simulink model "PMSM_SMO_dq"  (Simulink 9.3)
settings: Solver=ode3  StartTime=0.0  StopTime=1  FixedStep=Ts  RelTol=1e-3  EnableMultiTasking=on
InitFcn:
  | Ts = 10e-6;
  | 
  | Ra = 0.011;
  | Ld = 0.0016;
  | Lq = 0.001;
  | flux =0.077;
  | 
  | m0 = 2;
  | ksild = 700;
  | A = exp(-Ra/Ld*Ts);
  | B = (1-A)/Ra;
  | Aq = exp(-Ra/Lq*Ts);
  | Bq = (1-Aq)/Ra;
undefined symbols (not defined in the file or in its folder): DiscIntNeverNeededParam
libraries: powerlib_extras x9, powerlib x5, simulink x1
settings Model: Creator=Administrator  LastModifiedBy=Administrator
settings DataIOCC: LimitDataPoints=on
settings OptimizationCC: ExpressionDepthLimit=2147483647  InitFltsAndDblsToZero=on
settings DebuggingCC: SaveWithParameterizedLinksMsg=none  SolverPrmCheckMsg=warning  StateNameClashWarn=warning
settings GRTTargetCC: TargetFcnLib=ansi_tfl_tmw.mat  GeneratePreprocessorConditionals=Disable all
settings ConfigComp: CovSFcnEnable=off
settings SimscapeCC: SimscapeNormalizeSystem=off

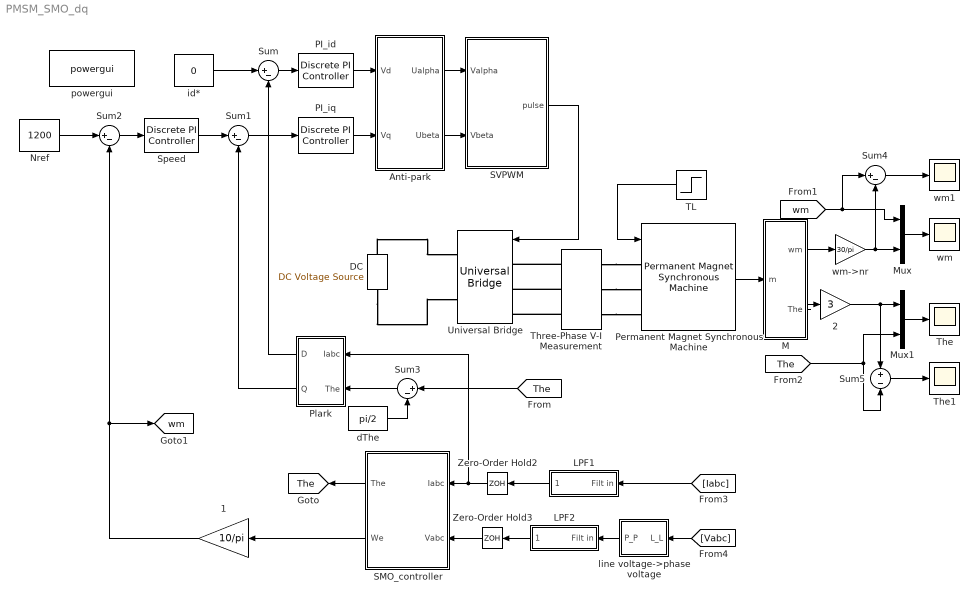
== system PMSM_SMO_dq ==
  1 : Gain  Gain=10/pi
  2 : Gain  Gain=3
  Anti-park : Subsystem
  "DC " : powerlib/Electrical Sources/DC Voltage Source  Amplitude=311  Measurements=None
      settings: SourceProductName=Simscape Electrical
  LPF1 : Subsystem  mask{wcc=3000, Ts=Ts}
      mask prompts: wcc "Control Filter cutoff frequency(Hz):"; Ts "sampling time"
  LPF2 : Subsystem  mask{wcc=3000, Ts=Ts}
      mask prompts: wcc "Control Filter cutoff frequency(Hz):"; Ts "sampling time"
  M : Subsystem
  Mux : Mux  Inputs=2
  Mux1 : Mux  Inputs=2
  Nref : Constant  Value=1200
  "PI_id " : powerlib_extras/Discrete  Control Blocks/Discrete PI Controller  Kp=0.0016*20000  Ki=0.011*20000  Par_Limits=[250 -250]  Init=0  Ts=Ts
      settings: SourceProductName=Simscape Electrical
  PI_iq : powerlib_extras/Discrete  Control Blocks/Discrete PI Controller  Kp=0.001*20000  Ki=0.011*20000  Par_Limits=[250 -250]  Init=0  Ts=Ts
      settings: SourceProductName=Simscape Electrical
  Permanent Magnet Synchronous Machine : powerlib/Machines/Permanent Magnet Synchronous Machine  NbPhases=3  FluxDistribution=Sinusoidal  RotorType=Salient-pole  MechanicalLoad=Torque Tm  PresetModel=No  ShowDetailedParameters=on  MeasurementBus=off  Resistance=0.011  Inductance=8.5e-3  dqInductances=[0.0016,0.001]  La=0.000835  MachineConstant=Flux linkage established by magnets (V.s)  Flux=0.077  VoltageCst=41.8988  TorqueCst=0.3465  Flat=120  Mechanical=[0.0008 0 3]  PolePairs=3  InitialConditions=[0,0, 0,0]  InitialConditions5ph=[0 0 0 0 0 0]  TsPowergui=0  TsBlock=-1  RefAngle=90 degrees behind phase A axis (modified Park)
  Plark : Subsystem
  SMO_controller : Subsystem  mask{Ts=Ts}
  SVPWM : Subsystem
  "Speed " : powerlib_extras/Discrete  Control Blocks/Discrete PI Controller  Kp=0.02  Ki=1  Par_Limits=[300 -300]  Init=0  Ts=Ts
      settings: SourceProductName=Simscape Electrical
  Sum{,1..4} (5 alike) : Sum  Inputs=|+-
  Sum5 : Sum  Inputs=+|-
  TL : Step  Time=0.5  After=1*0  SampleTime=0
  The : Scope
  The1 : Scope
  Three-Phase V-I Measurement : powerlib/Measurements/Three-Phase V-I Measurement  VoltageMeasurement=phase-to-phase  SetLabelV=on  LabelV=Vabc  Vpu=off  VpuLL=off  CurrentMeasurement=yes  SetLabelI=on  LabelI=Iabc  Ipu=off  Pbase=100e6  Vbase=500e3  OutputType=Complex  PhasorSimulation=off  PSBequivalent=0
      settings: SourceProductName=Simscape Electrical
  Universal Bridge : powerlib/Power Electronics/Universal Bridge  Arms=3  SnubberResistance=1e5  SnubberCapacitance=inf  Device=IGBT / Diodes  Ron=1e-3  Lon=0  ForwardVoltages="[  0  0  ]"  ForwardVoltage=0  GTOparameters=[ 10e-6 , 20e-6 ]  IGBTparameters=[ 1e-6 , 2e-6 ]  Measurements=None  Measurements_2=None  converterType=Rectifier
      settings: SourceProductName=Simscape Electrical
  Zero-Order Hold2 : ZeroOrderHold  SampleTime=Ts
  Zero-Order Hold3 : ZeroOrderHold  SampleTime=Ts
  dThe : Constant  Value=pi/2
  id* : Constant  Value=0
  line voltage->phase voltage : Subsystem
  powergui : powerlib/powergui  SimulationMode=Discrete  SampleTime=Ts  frequency=60  Iterations=50  frequencyindice=0  Pbase=100e6  ErrMax=1e-4  UnitsV=kV  UnitsW=MW  buscounter=0  FunctionMessages=off  echomessages=off  EnableUseOfTLC=off  CurrentSourceSwitches=off  DisableSnubberDevices=off  DisableRonSwitches=off  DisableVfSwitches=off  DisplayEquations=off  AutomaticDiscreteSolvers=off  SolverType=Tustin/Backward Euler (TBE)  Interpol=off  ExternalGateDelay=off  methode=off  Ts=0  x0status=blocks  SPID=off  SwTol=0  HookPort=off  NonlinearTolerance=0  nMaxIteration=15  ContinueOnMaxIteration=off  RestoreLinks=warning  ResistiveCurrentMeasurement=off  Frange=[0:2:500]  Ylog=off  Xlog=on  ShowGrid=off  save=off  variable=ZData  structure=0  ZoomFFT=off  StartTime=0.0  cycles=1  DisplayStyle=1  fundamental=60  FreqAxis=off  MaxFrequency=1000  frequencyindicesteady=1  RmsSteady=1  display=off
      settings: SourceProductName=Simscape Electrical
  wm : Scope
  wm->nr : Gain  Gain=30/pi
  wm1 : Scope
  tag scope: The=global, wm=global
  wires:
  SVPWM/1(pulse) -> Universal Bridge/1
  Permanent Magnet Synchronous Machine/1 -> M/1(m)
  "PI_id "/1 -> Anti-park/1(Vd)
  PI_iq/1 -> Anti-park/2(Vq)
  Sum/1 -> "PI_id "/1
  Sum1/1 -> PI_iq/1
  Sum2/1 -> "Speed "/1
  Nref/1 -> Sum2/1
  "Speed "/1 -> Sum1/1
  1/1 -> [wm], Sum2/2
  Anti-park/1(Ualpha) -> SVPWM/1(Valpha)
  Anti-park/2(Ubeta) -> SVPWM/2(Vbeta)
  TL/1 -> Permanent Magnet Synchronous Machine/1
  M/1(wm) -> wm->nr/1
  id*/1 -> Sum/1
  Plark/1(D) -> Sum/2
  Plark/2(Q) -> Sum1/2
  dThe/1 -> Sum3/2
  Sum3/1 -> Plark/2(The)
  M/2(The) -> 2/1
  LPF2/1(Filt out) -> Zero-Order Hold3/1
  Zero-Order Hold3/1 -> SMO_controller/2(Vabc)
  Zero-Order Hold2/1 -> Plark/1(Iabc), SMO_controller/1(Iabc)
  LPF1/1(Filt out) -> Zero-Order Hold2/1
  SMO_controller/1(The) -> [The]
  [The] -> Sum3/1
  wm->nr/1 -> Mux/2, Sum4/2
  [wm] -> Mux/1, Sum4/1
  Mux/1 -> wm/1
  Sum4/1 -> wm1/1
  2/1 -> Sum5/1, Mux1/1
  Mux1/1 -> The/1
  [The] -> Mux1/2, Sum5/2
  Sum5/1 -> The1/1
  [Iabc] -> LPF1/1(Filt in)
  [Vabc] -> line voltage->phase voltage/1(L_L)
  line voltage->phase voltage/1(P_P) -> LPF2/1(Filt in)
  SMO_controller/2(We) -> 1/1
  connections:
  "DC "/RConn1 -- Universal Bridge/RConn1
  "DC "/LConn1 -- Universal Bridge/RConn2
  Three-Phase V-I Measurement/LConn1 -- Universal Bridge/LConn1
  Three-Phase V-I Measurement/RConn1 -- Permanent Magnet Synchronous Machine/LConn1
  Three-Phase V-I Measurement/LConn2 -- Universal Bridge/LConn2
  Three-Phase V-I Measurement/LConn3 -- Universal Bridge/LConn3
  Three-Phase V-I Measurement/RConn2 -- Permanent Magnet Synchronous Machine/LConn2
  Three-Phase V-I Measurement/RConn3 -- Permanent Magnet Synchronous Machine/LConn3

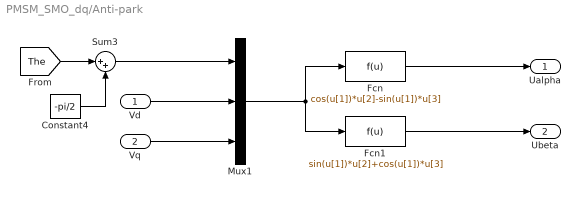
== system PMSM_SMO_dq/Anti-park ==
  Vd : Inport
  Vq : Inport  Port=2
  Constant4 : Constant  Value=-pi/2
  Fcn : Fcn  Expr=cos(u[1])*u[2]-sin(u[1])*u[3]
  Fcn1 : Fcn  Expr=sin(u[1])*u[2]+cos(u[1])*u[3]
  Mux1 : Mux  Inputs=3
  Sum3 : Sum  Inputs=|++
  Ualpha : Outport
  Ubeta : Outport  Port=2
  wires:
  Fcn1/1 -> Ubeta/1
  Fcn/1 -> Ualpha/1
  Mux1/1 -> Fcn/1, Fcn1/1
  Vd/1 -> Mux1/2
  Vq/1 -> Mux1/3
  Sum3/1 -> Mux1/1
  [The] -> Sum3/1
  Constant4/1 -> Sum3/2

== system PMSM_SMO_dq/LPF1 ==
  Filt in : Inport
  Demux1 : Demux  Outputs=3
  LPF1 : powerlib_extras/Discrete  Control Blocks/Discrete 1st-Order Filter  FilterType=Lowpass  Tc=1/(2*pi*wcc)  Ts=Ts  Initialize=off  Vac_Init=[0.8 -25 60]  Vdc_Init=-0.4  PlotResponse=off  param1=[1 500 1]
      settings: SourceProductName=Simscape Electrical  SourceProductBaseCode=PS
  LPF2 : powerlib_extras/Discrete  Control Blocks/Discrete 1st-Order Filter  FilterType=Lowpass  Tc=1/(2*pi*wcc)  Ts=Ts  Initialize=off  Vac_Init=[0.8 -25 60]  Vdc_Init=-0.4  PlotResponse=off  param1=[1 500 1]
      settings: SourceProductName=Simscape Electrical  SourceProductBaseCode=PS
  LPF3 : powerlib_extras/Discrete  Control Blocks/Discrete 1st-Order Filter  FilterType=Lowpass  Tc=1/(2*pi*wcc)  Ts=Ts  Initialize=off  Vac_Init=[0.8 -25 60]  Vdc_Init=-0.4  PlotResponse=off  param1=[1 4000 1]
      settings: SourceProductName=Simscape Electrical  SourceProductBaseCode=PS
  Mux1 : Mux  Inputs=3
  Filt out : Outport
  wires:
  Demux1/1 -> LPF1/1
  LPF1/1 -> Mux1/1
  Demux1/2 -> LPF2/1
  LPF2/1 -> Mux1/2
  Filt in/1 -> Demux1/1
  Mux1/1 -> Filt out/1
  Demux1/3 -> LPF3/1
  LPF3/1 -> Mux1/3

== system PMSM_SMO_dq/LPF2 ==
  Filt in : Inport
  Demux1 : Demux  Outputs=3
  LPF1 : powerlib_extras/Discrete  Control Blocks/Discrete 1st-Order Filter  FilterType=Lowpass  Tc=1/(2*pi*wcc)  Ts=Ts  Initialize=off  Vac_Init=[0.8 -25 60]  Vdc_Init=-0.4  PlotResponse=off  param1=[1 500 1]
      settings: SourceProductName=Simscape Electrical  SourceProductBaseCode=PS
  LPF2 : powerlib_extras/Discrete  Control Blocks/Discrete 1st-Order Filter  FilterType=Lowpass  Tc=1/(2*pi*wcc)  Ts=Ts  Initialize=off  Vac_Init=[0.8 -25 60]  Vdc_Init=-0.4  PlotResponse=off  param1=[1 500 1]
      settings: SourceProductName=Simscape Electrical  SourceProductBaseCode=PS
  LPF3 : powerlib_extras/Discrete  Control Blocks/Discrete 1st-Order Filter  FilterType=Lowpass  Tc=1/(2*pi*wcc)  Ts=Ts  Initialize=off  Vac_Init=[0.8 -25 60]  Vdc_Init=-0.4  PlotResponse=off  param1=[1 4000 1]
      settings: SourceProductName=Simscape Electrical  SourceProductBaseCode=PS
  Mux1 : Mux  Inputs=3
  Filt out : Outport
  wires:
  LPF3/1 -> Mux1/3
  Demux1/3 -> LPF3/1
  Mux1/1 -> Filt out/1
  Filt in/1 -> Demux1/1
  LPF2/1 -> Mux1/2
  Demux1/2 -> LPF2/1
  LPF1/1 -> Mux1/1
  Demux1/1 -> LPF1/1

== system PMSM_SMO_dq/M ==
  m : Inport
  Bus Selector1 : BusSelector  OutputSignals=Rotor speed wm (rad/s),Rotor angle thetam (rad),Electromagnetic torque Te (N*m)
  Terminator : Terminator
  wm : Outport
  The : Outport  Port=2
  wires:
  Bus Selector1/1 -> wm/1  "<Rotor speed wm (rad/s)>"
  Bus Selector1/2 -> The/1  "<Rotor angle thetam (rad)>"
  Bus Selector1/3 -> Terminator/1  "<Electromagnetic torque Te (N*m)>"
  m/1 -> Bus Selector1/1

== system PMSM_SMO_dq/Plark ==
  Iabc : Inport
  The : Inport  Port=2
  Mux : Mux  Inputs=2
  d : Fcn  Expr=(u(1)*cos(u(4))+u(2)*cos(u(4)-2/3*pi)+u(3)*cos(u(4)+2/3*pi))*2/3
  q : Fcn  Expr=-(u(1)*sin(u(4))+u(2)*sin(u(4)-2/3*pi)+u(3)*sin(u(4)+2/3*pi))*2/3
  D : Outport
  Q : Outport  Port=2
  wires:
  Mux/1 -> d/1, q/1
  Iabc/1 -> Mux/1
  d/1 -> D/1
  The/1 -> Mux/2
  q/1 -> Q/1

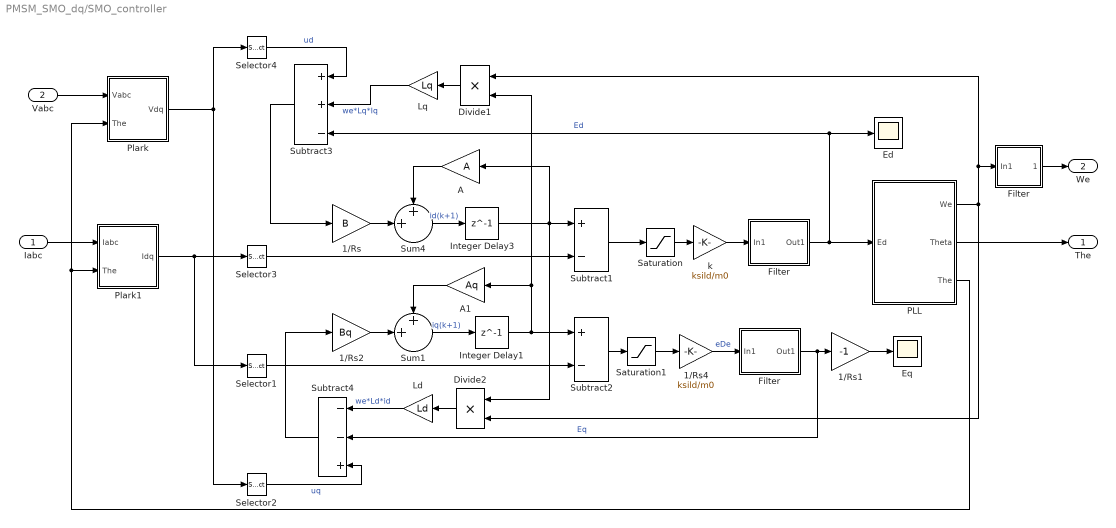
== system PMSM_SMO_dq/SMO_controller ==
  Iabc : Inport
  Vabc : Inport  Port=2
  " Filter" : Subsystem  mask{a=0.97}
  1/Rs : Gain  Gain=B
  1/Rs1 : Gain  Gain=-1
  1/Rs2 : Gain  Gain=Bq
  1/Rs4 : Gain  Gain=ksild/m0
  A : Gain  Gain=A
  A1 : Gain  Gain=Aq
  Divide1 : Product  Inputs=**
  Divide2 : Product  Inputs=**
  Ed : Scope
  Eq : Scope
  "Filter " : Subsystem  mask{a=0.97}
  "Filter  " : Subsystem  mask{a=0.99}
  Integer Delay1 : Delay  DelayLength=1  SampleTime=Ts
  Integer Delay3 : Delay  DelayLength=1  SampleTime=Ts
  Ld : Gain  Gain=Ld
  Lq : Gain  Gain=Lq
  PLL : Subsystem
  Plark : Subsystem
  Plark1 : Subsystem
  Saturation : Saturate  UpperLimit=m0  LowerLimit=-m0
  Saturation1 : Saturate  UpperLimit=m0  LowerLimit=-m0
  Selector1 : Selector  InputPortWidth=2  IndexOptions=Index vector (dialog)  Indices=[2 ]  OutputSizes=1
  Selector2 : Selector  InputPortWidth=2  IndexOptions=Index vector (dialog)  Indices=[2 ]  OutputSizes=1
  Selector3 : Selector  InputPortWidth=2  IndexOptions=Index vector (dialog)  Indices=[1 ]  OutputSizes=1
  Selector4 : Selector  InputPortWidth=2  IndexOptions=Index vector (dialog)  Indices=[1 ]  OutputSizes=1
  Subtract1 : Sum  Inputs=+-
  Subtract2 : Sum  Inputs=+-
  Subtract3 : Sum  Inputs=++-
  Subtract4 : Sum  Inputs=--+
  Sum1 : Sum  Inputs=++|
  Sum4 : Sum  Inputs=++|
  k : Gain  Gain=ksild/m0
  The : Outport
  We : Outport  Port=2
  wires:
  Iabc/1 -> Plark1/1(Iabc)
  Vabc/1 -> Plark/1(Vabc)
  Plark1/1(Idq) -> Selector1/1, Selector3/1
  Plark/1(Vdq) -> Selector4/1, Selector2/1
  Lq/1 -> Subtract3/2  "we*Lq*Iq"
  Saturation/1 -> k/1
  Divide1/1 -> Lq/1
  Sum4/1 -> Integer Delay3/1  "id(k+1)"
  Subtract1/1 -> Saturation/1
  k/1 -> "Filter "/1(In1)
  Subtract3/1 -> 1/Rs/1
  Selector4/1 -> Subtract3/1  "ud"
  1/Rs/1 -> Sum4/2
  A/1 -> Sum4/1
  Selector3/1 -> Subtract1/2
  "Filter "/1(Out1) -> Ed/1, Subtract3/3, PLL/1(Ed)  "Ed"
  Saturation1/1 -> 1/Rs4/1
  Divide2/1 -> Ld/1
  Sum1/1 -> Integer Delay1/1  "iq(k+1)"
  Subtract2/1 -> Saturation1/1
  1/Rs4/1 -> " Filter"/1(In1)  "eDe"
  Subtract4/1 -> 1/Rs2/1
  1/Rs2/1 -> Sum1/2
  " Filter"/1(Out1) -> 1/Rs1/1, Subtract4/2  "Eq"
  A1/1 -> Sum1/1
  Selector1/1 -> Subtract2/2
  Integer Delay1/1 -> Subtract2/1, Divide1/2, A1/1
  Ld/1 -> Subtract4/1  "we*Ld*id"
  Selector2/1 -> Subtract4/3  "uq"
  Integer Delay3/1 -> Subtract1/1, A/1, Divide2/1
  PLL/3(The) -> Plark/2(The), Plark1/2(The)
  PLL/1(We) -> Divide1/1, "Filter  "/1(In1), Divide2/2
  PLL/2(Theta) -> The/1
  "Filter  "/1(Out1) -> We/1
  1/Rs1/1 -> Eq/1

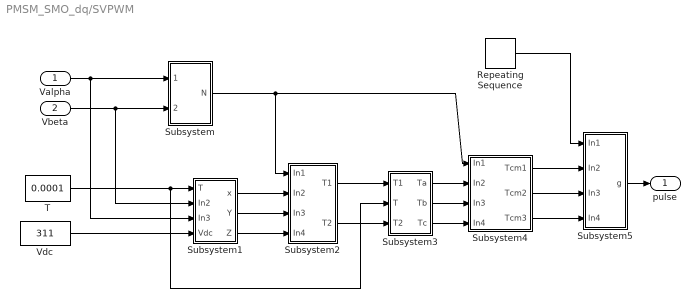
== system PMSM_SMO_dq/SVPWM ==
  Valpha : Inport
  Vbeta : Inport  Port=2
  Repeating Sequence : simulink/Sources/Repeating Sequence  rep_seq_t=[0 0.00005 0.0001]  rep_seq_y=[0 0.00005 0]
  Subsystem : Subsystem
  Subsystem1 : Subsystem
  Subsystem2 : Subsystem
  Subsystem3 : Subsystem
  Subsystem4 : Subsystem
  Subsystem5 : Subsystem
  T : Constant  Value=0.0001
  Vdc : Constant  Value=311
  pulse : Outport
  wires:
  Subsystem5/1(g) -> pulse/1
  Repeating Sequence/1 -> Subsystem5/1(In1)
  Subsystem4/3(Tcm3) -> Subsystem5/4(In4)
  Subsystem4/2(Tcm2) -> Subsystem5/3(In3)
  Subsystem4/1(Tcm1) -> Subsystem5/2(In2)
  Subsystem3/3(Tc) -> Subsystem4/4(In4)
  Subsystem3/2(Tb) -> Subsystem4/3(In3)
  Subsystem3/1(Ta) -> Subsystem4/2(In2)
  Subsystem2/2(T2) -> Subsystem3/3(T2)
  Subsystem2/1(T1) -> Subsystem3/1(T1)
  Subsystem1/3(Z) -> Subsystem2/4(In4)
  Subsystem1/2(Y) -> Subsystem2/3(In3)
  Subsystem1/1(x) -> Subsystem2/2(In2)
  Subsystem/1(N) -> Subsystem4/1(In1), Subsystem2/1(In1)
  Vdc/1 -> Subsystem1/4(Vdc)
  T/1 -> Subsystem3/2(T), Subsystem1/1(T)
  Vbeta/1 -> Subsystem1/2(In2), Subsystem/2(Vbeta)
  Valpha/1 -> Subsystem1/3(In3), Subsystem/1(Valpha)

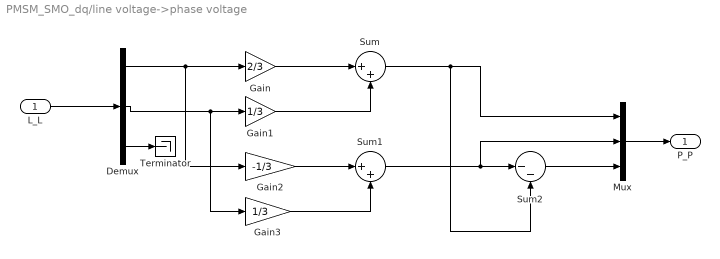
== system PMSM_SMO_dq/line voltage->phase voltage ==
  L_L : Inport
  Demux : Demux  Outputs=3
  Gain : Gain  Gain=2/3
  Gain1 : Gain  Gain=1/3
  Gain2 : Gain  Gain=-1/3
  Gain3 : Gain  Gain=1/3
  Mux : Mux  Inputs=3
  Sum : Sum  Inputs=|++
  Sum1 : Sum  Inputs=|++
  Sum2 : Sum  Inputs=|--
  Terminator : Terminator
  P_P : Outport
  wires:
  Demux/2 -> Gain3/1, Gain1/1
  Demux/1 -> Gain2/1, Gain/1
  Gain/1 -> Sum/1
  Gain1/1 -> Sum/2
  Gain2/1 -> Sum1/1
  Gain3/1 -> Sum1/2
  Sum/1 -> Sum2/2, Mux/1
  Sum2/1 -> Mux/3
  Sum1/1 -> Mux/2, Sum2/1
  Mux/1 -> P_P/1
  L_L/1 -> Demux/1
  Demux/3 -> Terminator/1

== system PMSM_SMO_dq/SMO_controller/ Filter ==
  In1 : Inport
  1/Ld1 : Gain  Gain=a
  1/Ld4 : Gain  Gain=1-a  SampleTime=Ts
  Integer Delay5 : Delay  DelayLength=1  SampleTime=Ts
  Subtract3 : Sum
  Out1 : Outport
  wires:
  In1/1 -> 1/Ld4/1
  1/Ld1/1 -> Subtract3/2
  1/Ld4/1 -> Subtract3/1
  Integer Delay5/1 -> 1/Ld1/1
  Subtract3/1 -> Out1/1, Integer Delay5/1

== system PMSM_SMO_dq/SMO_controller/Filter  ==
  In1 : Inport
  1/Ld1 : Gain  Gain=a
  1/Ld4 : Gain  Gain=1-a  SampleTime=Ts
  Integer Delay5 : Delay  DelayLength=1  SampleTime=Ts
  Subtract3 : Sum
  Out1 : Outport
  wires:
  In1/1 -> 1/Ld4/1
  1/Ld1/1 -> Subtract3/2
  1/Ld4/1 -> Subtract3/1
  Integer Delay5/1 -> 1/Ld1/1
  Subtract3/1 -> Out1/1, Integer Delay5/1

== system PMSM_SMO_dq/SMO_controller/Filter   ==
  In1 : Inport
  1/Ld1 : Gain  Gain=a
  1/Ld4 : Gain  Gain=1-a  SampleTime=Ts
  Integer Delay5 : Delay  DelayLength=1  SampleTime=Ts
  Subtract3 : Sum
  Out1 : Outport
  wires:
  Subtract3/1 -> Integer Delay5/1, Out1/1
  Integer Delay5/1 -> 1/Ld1/1
  1/Ld4/1 -> Subtract3/1
  1/Ld1/1 -> Subtract3/2
  In1/1 -> 1/Ld4/1

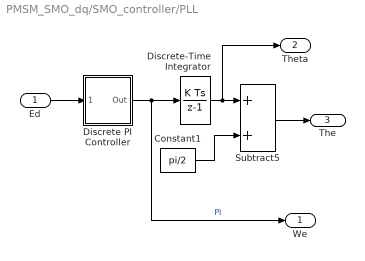
== system PMSM_SMO_dq/SMO_controller/PLL ==
  Ed : Inport
  Constant1 : Constant  Value=pi/2
  Discrete PI Controller : Subsystem  AncestorBlock=|  mask(Discrete PI Controller){Kp=30, Ki=225*2, Par_Limits=[1000 -1000], Init=0, Ts=Ts}
      | powerlib_extras/Discrete 
      | Control Blocks/Discrete
      | PI Controller
      mask prompts: Kp "Proportional gain (Kp):"; Ki "Integral gain (Ki):"; Par_Limits "Output limits: [ Upper   Lower ]"; Init "Output initial value:"; Ts "Sample time:"
      mask help: This block implements a discrete PI controller.
      mask init:
      | UpperLimit=Par_Limits(1);
      | LowerLimit=Par_Limits(2);
      | power_initmask();
      settings: OpenFcn=power_openblockproxy();
      mask Display: disp('PI');
  Discrete-Time Integrator : DiscreteIntegrator  SampleTime=Ts  ICPrevOutput=DiscIntNeverNeededParam  ICPrevScaledInput=DiscIntNeverNeededParam
  Subtract5 : Sum
  We : Outport
  Theta : Outport  Port=2
  The : Outport  Port=3
  wires:
  Discrete-Time Integrator/1 -> Theta/1, Subtract5/1
  Subtract5/1 -> The/1
  Constant1/1 -> Subtract5/2
  Discrete PI Controller/1(Out) -> We/1, Discrete-Time Integrator/1  "PI"
  Ed/1 -> Discrete PI Controller/1(Error)

== system PMSM_SMO_dq/SMO_controller/Plark ==
  Vabc : Inport
  The : Inport  Port=2
  Mux : Mux  Inputs=2
  Mux1 : Mux  Inputs=2
  d : Fcn  Expr=(u(1)*cos(u(4))+u(2)*cos(u(4)-2/3*pi)+u(3)*cos(u(4)+2/3*pi))*2/3
  q : Fcn  Expr=-(u(1)*sin(u(4))+u(2)*sin(u(4)-2/3*pi)+u(3)*sin(u(4)+2/3*pi))*2/3
  Vdq : Outport
  wires:
  Mux/1 -> q/1, d/1
  Vabc/1 -> Mux/1
  The/1 -> Mux/2
  d/1 -> Mux1/1
  q/1 -> Mux1/2
  Mux1/1 -> Vdq/1

== system PMSM_SMO_dq/SMO_controller/Plark1 ==
  Iabc : Inport
  The : Inport  Port=2
  Mux : Mux  Inputs=2
  Mux1 : Mux  Inputs=2
  d : Fcn  Expr=(u(1)*cos(u(4))+u(2)*cos(u(4)-2/3*pi)+u(3)*cos(u(4)+2/3*pi))*2/3
  q : Fcn  Expr=-(u(1)*sin(u(4))+u(2)*sin(u(4)-2/3*pi)+u(3)*sin(u(4)+2/3*pi))*2/3
  Idq : Outport
  wires:
  Mux1/1 -> Idq/1
  q/1 -> Mux1/2
  d/1 -> Mux1/1
  The/1 -> Mux/2
  Iabc/1 -> Mux/1
  Mux/1 -> d/1, q/1

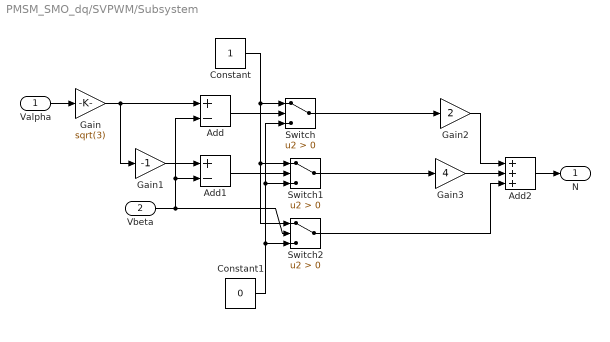
== system PMSM_SMO_dq/SVPWM/Subsystem ==
  Valpha : Inport
  Vbeta : Inport  Port=2
  Add : Sum  Inputs=+-
  Add1 : Sum  Inputs=+-
  Add2 : Sum  Inputs=+++
  Constant : Constant
  Constant1 : Constant  Value=0
  Gain : Gain  Gain=sqrt(3)
  Gain1 : Gain  Gain=-1
  Gain2 : Gain  Gain=2
  Gain3 : Gain  Gain=4
  Switch : Switch  Criteria=u2 > Threshold
  Switch1 : Switch  Criteria=u2 > Threshold
  Switch2 : Switch  Criteria=u2 > Threshold
  N : Outport
  wires:
  Add2/1 -> N/1
  Valpha/1 -> Gain/1
  Gain3/1 -> Add2/2
  Gain2/1 -> Add2/1
  Add1/1 -> Switch1/2
  Gain1/1 -> Add1/1
  Switch1/1 -> Gain3/1
  Switch2/1 -> Add2/3
  Switch/1 -> Gain2/1
  Add/1 -> Switch/2
  Gain/1 -> Gain1/1, Add/1
  Constant1/1 -> Switch/3, Switch1/3, Switch2/3
  Constant/1 -> Switch1/1, Switch2/1, Switch/1
  Vbeta/1 -> Add1/2, Add/2, Switch2/2

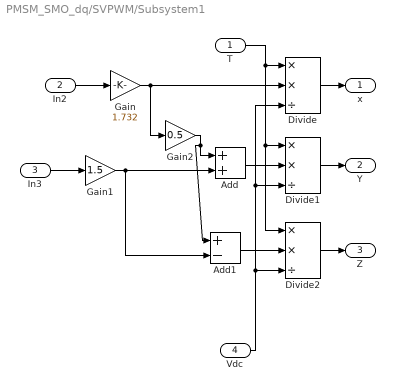
== system PMSM_SMO_dq/SVPWM/Subsystem1 ==
  T : Inport
  In2 : Inport  Port=2
  In3 : Inport  Port=3
  Vdc : Inport  Port=4
  Add : Sum
  Add1 : Sum  Inputs=+-
  Divide : Product  Inputs=**/
  Divide1 : Product  Inputs=**/
  Divide2 : Product  Inputs=**/
  Gain : Gain  Gain=1.732
  Gain1 : Gain  Gain=1.5
  Gain2 : Gain  Gain=0.5
  x : Outport
  Y : Outport  Port=2
  Z : Outport  Port=3
  wires:
  Divide2/1 -> Z/1
  Divide1/1 -> Y/1
  Divide/1 -> x/1
  In3/1 -> Gain1/1
  In2/1 -> Gain/1
  Add1/1 -> Divide2/2
  Add/1 -> Divide1/2
  Gain1/1 -> Add1/2, Add/2
  Gain2/1 -> Add1/1, Add/1
  Gain/1 -> Gain2/1, Divide/2
  Vdc/1 -> Divide/3, Divide1/3, Divide2/3
  T/1 -> Divide2/1, Divide1/1, Divide/1

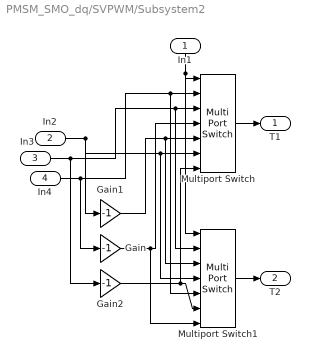
== system PMSM_SMO_dq/SVPWM/Subsystem2 ==
  In1 : Inport
  In2 : Inport  Port=2
  In3 : Inport  Port=3
  In4 : Inport  Port=4
  Gain : Gain  Gain=-1
  Gain1 : Gain  Gain=-1
  Gain2 : Gain  Gain=-1
  Multiport Switch : MultiPortSwitch  Inputs=6
  Multiport Switch1 : MultiPortSwitch  Inputs=6
  T1 : Outport
  T2 : Outport  Port=2
  wires:
  Multiport Switch1/1 -> T2/1
  Multiport Switch/1 -> T1/1
  Gain2/1 -> Multiport Switch/7, Multiport Switch1/6
  Gain1/1 -> Multiport Switch1/3, Multiport Switch/5
  In2/1 -> Gain1/1, Multiport Switch/6, Multiport Switch1/4
  Gain/1 -> Multiport Switch1/7, Multiport Switch/4
  In3/1 -> Gain2/1, Multiport Switch1/2, Multiport Switch/3
  In4/1 -> Gain/1, Multiport Switch/2, Multiport Switch1/5
  In1/1 -> Multiport Switch/1, Multiport Switch1/1

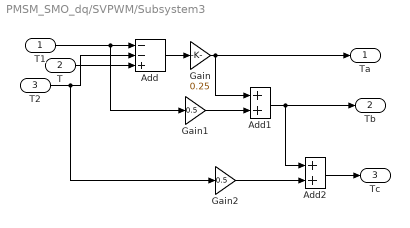
== system PMSM_SMO_dq/SVPWM/Subsystem3 ==
  T1 : Inport
  T : Inport  Port=2
  T2 : Inport  Port=3
  Add : Sum  Inputs=--+
  Add1 : Sum
  Add2 : Sum
  Gain : Gain  Gain=0.25
  Gain1 : Gain  Gain=0.5
  Gain2 : Gain  Gain=0.5
  Ta : Outport
  Tb : Outport  Port=2
  Tc : Outport  Port=3
  wires:
  T/1 -> Add/3
  Add2/1 -> Tc/1
  Gain2/1 -> Add2/2
  Add1/1 -> Add2/1, Tb/1
  Gain1/1 -> Add1/2
  Gain/1 -> Add1/1, Ta/1
  Add/1 -> Gain/1
  T2/1 -> Add/2, Gain2/1
  T1/1 -> Add/1, Gain1/1

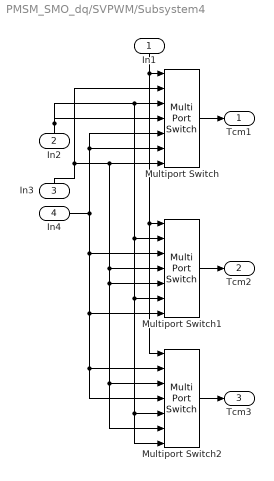
== system PMSM_SMO_dq/SVPWM/Subsystem4 ==
  In1 : Inport
  In2 : Inport  Port=2
  In3 : Inport  Port=3
  In4 : Inport  Port=4
  Multiport Switch : MultiPortSwitch  Inputs=6
  Multiport Switch1 : MultiPortSwitch  Inputs=6
  Multiport Switch2 : MultiPortSwitch  Inputs=6
  Tcm1 : Outport
  Tcm2 : Outport  Port=2
  Tcm3 : Outport  Port=3
  wires:
  Multiport Switch2/1 -> Tcm3/1
  Multiport Switch1/1 -> Tcm2/1
  Multiport Switch/1 -> Tcm1/1
  In1/1 -> Multiport Switch2/1, Multiport Switch1/1, Multiport Switch/1
  In4/1 -> Multiport Switch1/3, Multiport Switch1/7, Multiport Switch2/2, Multiport Switch2/4, Multiport Switch/5, Multiport Switch/6
  In2/1 -> Multiport Switch/4, Multiport Switch/3, Multiport Switch1/2, Multiport Switch1/6, Multiport Switch2/5, Multiport Switch2/7
  In3/1 -> Multiport Switch/2, Multiport Switch/7, Multiport Switch1/4, Multiport Switch1/5, Multiport Switch2/3, Multiport Switch2/6

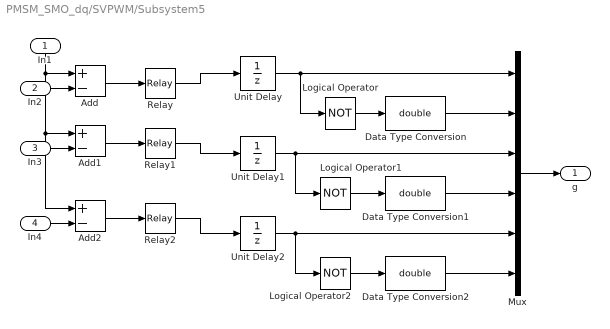
== system PMSM_SMO_dq/SVPWM/Subsystem5 ==
  In1 : Inport
  In2 : Inport  Port=2
  In3 : Inport  Port=3
  In4 : Inport  Port=4
  Add : Sum  Inputs=+-
  Add1 : Sum  Inputs=+-
  Add2 : Sum  Inputs=+-
  Data Type Conversion : DataTypeConversion  OutDataTypeStr=double
  Data Type Conversion1 : DataTypeConversion  OutDataTypeStr=double
  Data Type Conversion2 : DataTypeConversion  OutDataTypeStr=double
  Logical Operator : Logic  Operator=NOT  AllPortsSameDT=off  OutDataTypeStr=boolean
  Logical Operator1 : Logic  Operator=NOT  AllPortsSameDT=off  OutDataTypeStr=boolean
  Logical Operator2 : Logic  Operator=NOT  AllPortsSameDT=off  OutDataTypeStr=boolean
  Mux : Mux  Inputs=6
  Relay : Relay  OffSwitchValue=-eps
  Relay1 : Relay  OffSwitchValue=-eps
  Relay2 : Relay  OffSwitchValue=-eps
  Unit Delay : UnitDelay  SampleTime=-1  HasFrameUpgradeWarning=on
  Unit Delay1 : UnitDelay  SampleTime=-1  HasFrameUpgradeWarning=on
  Unit Delay2 : UnitDelay  SampleTime=-1  HasFrameUpgradeWarning=on
  g : Outport
  wires:
  In4/1 -> Add2/2
  In3/1 -> Add1/2
  In2/1 -> Add/2
  Relay2/1 -> Unit Delay2/1
  Relay1/1 -> Unit Delay1/1
  Relay/1 -> Unit Delay/1
  Unit Delay2/1 -> Mux/5, Logical Operator2/1
  Unit Delay1/1 -> Mux/3, Logical Operator1/1
  Unit Delay/1 -> Logical Operator/1, Mux/1
  Mux/1 -> g/1
  Data Type Conversion/1 -> Mux/2
  Data Type Conversion1/1 -> Mux/4
  Data Type Conversion2/1 -> Mux/6
  Logical Operator2/1 -> Data Type Conversion2/1
  Logical Operator1/1 -> Data Type Conversion1/1
  Logical Operator/1 -> Data Type Conversion/1
  Add1/1 -> Relay1/1
  Add2/1 -> Relay2/1
  Add/1 -> Relay/1
  In1/1 -> Add/1, Add2/1, Add1/1

== system PMSM_SMO_dq/SMO_controller/PLL/Discrete PI Controller ==
  note: Discrete PID Controller
  note: Pierre Giroux, Gilbert Sybille
      | Power System Simulation Laboratory
      | IREQ, Hydro-Quebc
  Error : Inport
  Discrete-Time Integrator : DiscreteIntegrator  SampleTime=Ts  LimitOutput=on  UpperSaturationLimit=UpperLimit  LowerSaturationLimit=LowerLimit  ICPrevOutput=DiscIntNeverNeededParam  ICPrevScaledInput=DiscIntNeverNeededParam
  Kp4 : Gain  Gain=Kp  SaturateOnIntegerOverflow=on  OutDataTypeStr=Inherit: Same as input  ParamDataTypeStr=Inherit: Same as input
  Kp5 : Gain  Gain=Ki  SaturateOnIntegerOverflow=on  OutDataTypeStr=Inherit: Same as input  ParamDataTypeStr=Inherit: Same as input
  Saturation2 : Saturate  UpperLimit=UpperLimit  LowerLimit=LowerLimit
  Sum6 : Sum  SaturateOnIntegerOverflow=on  InputSameDT=on  OutDataTypeStr=Inherit: Same as first input
  Out : Outport  InitialOutput=0
  wires:
  Saturation2/1 -> Out/1
  Discrete-Time Integrator/1 -> Sum6/2
  Kp4/1 -> Sum6/1
  Kp5/1 -> Discrete-Time Integrator/1
  Sum6/1 -> Saturation2/1
  Error/1 -> Kp5/1, Kp4/1
